simulink model "Pacemaker"  (R2020a)
settings: Solver=FixedStepAuto  StartTime=0.0  StopTime=10.0  FixedStep=1e-3  RelTol=1e-3  EnableMultiTasking=on
undefined symbols (not defined in the file or in its folder): A0, A1, D0, D1, D10, D11, D12, D13, D2, D3, D4, D5, D6, D7, D8, D9, PTA0, PTA1, PTA2, PTB2, PTB23, PTB3, PTB9, PTC16, PTC17, PTC2, PTC3, PTC4, PTD0, PTD1, PTD2, PTD3
libraries: frdmk64flib x21, etargetslib x12, simulink x2
settings Model: ExtModeTrigDuration=5  Creator=Udeep  LastModifiedBy=Udeep
settings OptimizationCC: EnhancedBackFolding=on  PassReuseOutputArgsAs=Individual arguments  ZeroExternalMemoryAtStartup=off  ZeroInternalMemoryAtStartup=off  MaxStackSize=64  OptimizeBlockOrder=speed  DifferentSizesBufferReuse=on  OptimizationCustomize=off  EfficientTunableParamExpr=on
settings DebuggingCC: ParameterTunabilityLossMsg=error
settings HardwareCC: ProdBitPerPointer=32  ProdBitPerSizeT=32  ProdBitPerPtrDiffT=32  ProdLargestAtomicInteger=Long  ProdLargestAtomicFloat=Double  ProdWordSize=32  ProdHWDeviceType=ARM Compatible->ARM Cortex
settings SFSimCC: MATLABDynamicMemAlloc=off
settings RTWCC: SystemTargetFile=ert.tlc  HardwareBoard=NXP FRDM-K64F  TemplateMakefile=ert_default_tmf  Toolchain=GNU Tools for ARM Embedded Processors
settings CodeAppCC: ForceParamTrailComments=on  IgnoreCustomStorageClasses=off  OperatorAnnotations=on  SimulinkDataObjDesc=on  SFDataObjDesc=on  InsertBlockDesc=on
settings ERTTargetCC: TargetLangStandard=C99 (ISO)

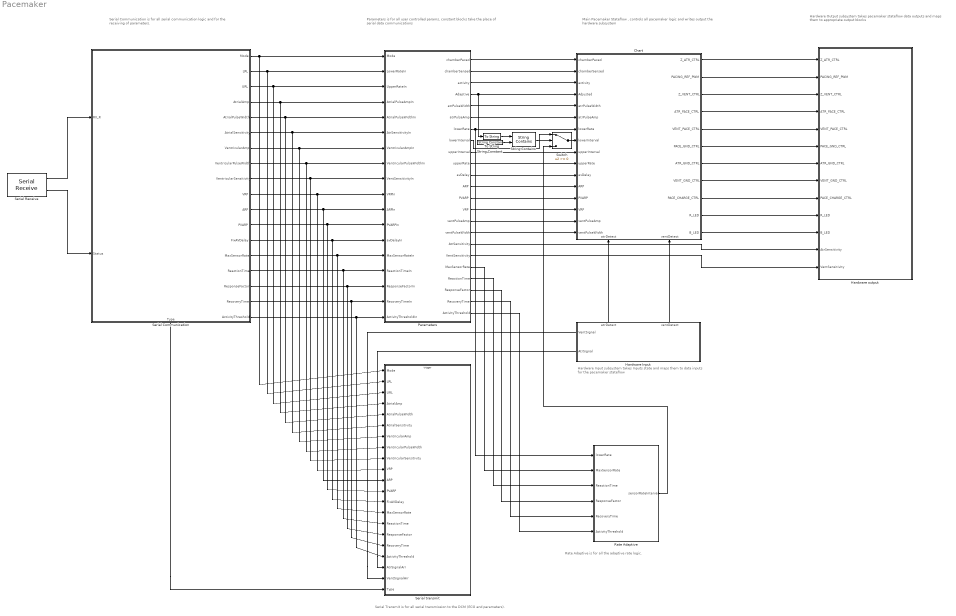
== system Pacemaker ==
  note: Hardware Input subsystem takes Inputs state and maps them to data inputs for the pacemaker stateflow
  note: Hardware Output subsystem takes pacemaker stateflow data outputs and maps them to appropriate output blocks
  note: Main Pacemaker Stateflow , controls all pacemaker logic and writes output the hardware subsystem
  note: Parameters is for all user controlled params, constant blocks take the place of serial data communications
  note: Serial Communication is for all serial communication logic and for the receiving of parameters.
  note: Serial Transmit is for all serial transmission to the DCM (ECG and parameters).
  note: Rate Adaptive is for all the adaptive rate logic.
  Chart : Stateflow chart  TreatAsAtomicUnit=on
      settings: PortSchema="{\"entries\":[{\"content\":{\"sides\":[{\"content\":{\"connectorIds\":[\"In4\",\"In6\",\"In7\",\"In5\",\"In8\",\"In9\",\"In17\",\"In10\",\"In11\",\"In18\",\"In12\",\"In13\",\"In16\",\"In1\",\"In14\",\"In15\"]},\"type\":\"ConnectorPlacement.EquallySpacedRectSide\",\"uuid\":\"0f4bb13e-4f4f-48e2-b63c-32132ec29449\"},{\"content\":{\"connectorIds\":[\"Out1\",\"Out2\",\"Out3\",\"Out4\",\"Out5\",\"Out6\",\"Out7\",\"Out8\",\"Out9\",\"Out10\",\"Out11\"],\"side\":\"RIGHT\"},\"type\":\"ConnectorPlacement.EquallySpacedRectSide\",\"uuid\":\"66676ed7-b2a9-4718-87b6-7ef1563d11ef\"},{\"content\":{\"connectorIds\":[],\"side\":\"TOP\"},\"type\":\"ConnectorPlacement.EquallySpacedRectSide\",\"uuid\":\"f8ed3d2c-017d-4860-9941-e982831d4406\"},{\"content\":{\"connectorIds\":[\"In2\",\"In3\"],\"side\":\"BOTTOM\"},\"type\":\"ConnectorPlacement.EquallySpacedRectSide\",\"uuid\":\"e6b63469-3180-4838-a33b-c03ead75d417\"}]},\"type\":\"ConnectorPlacement.EquallySpacedConnector\",\"uuid\":\"d1db759d-e7ed-4d4b-bc59-5cab093840d4\"}],\"packageUris\":[\"http://schema.mathworks.com/mf0/Connector/19700101\"],\"version\":\"1.0\"}"
  "Hardware Input " : Subsystem
      settings: PortSchema="{\"entries\":[{\"content\":{\"sides\":[{\"content\":{\"connectorIds\":[\"Out3\",\"Out4\"]},\"type\":\"ConnectorPlacement.EquallySpacedRectSide\",\"uuid\":\"9a02dc5a-1337-49ab-8682-c00d401b1034\"},{\"content\":{\"connectorIds\":[],\"side\":\"RIGHT\"},\"type\":\"ConnectorPlacement.EquallySpacedRectSide\",\"uuid\":\"4abd6ab8-13f7-4ac3-81e8-def358981a0b\"},{\"content\":{\"connectorIds\":[\"Out1\",\"Out2\"],\"side\":\"TOP\"},\"type\":\"ConnectorPlacement.EquallySpacedRectSide\",\"uuid\":\"0229585c-8215-4d3e-817f-7000ac7de4ec\"}]},\"type\":\"ConnectorPlacement.EquallySpacedConnector\",\"uuid\":\"98513f05-3720-42c8-8b88-fad36926c18f\"}],\"packageUris\":[\"http://schema.mathworks.com/mf0/Connector/19700101\"],\"version\":\"1.0\"}"
  Hardware output : Subsystem
  Parameters : Subsystem
  Rate Adaptive : Subsystem
  Serial Communication : Stateflow chart  TreatAsAtomicUnit=on
      settings: PortSchema="{\"entries\":[{\"content\":{\"sides\":[{\"content\":{\"connectorIds\":[\"In1\",\"In2\"]},\"type\":\"ConnectorPlacement.EquallySpacedRectSide\",\"uuid\":\"7ad26d3d-dec4-4b7e-9b47-df96273e8372\"},{\"content\":{\"connectorIds\":[\"Out1\",\"Out2\",\"Out3\",\"Out4\",\"Out5\",\"Out16\",\"Out6\",\"Out7\",\"Out17\",\"Out8\",\"Out9\",\"Out10\",\"Out11\",\"Out12\",\"Out13\",\"Out14\",\"Out15\",\"Out18\"],\"side\":\"RIGHT\"},\"type\":\"ConnectorPlacement.EquallySpacedRectSide\",\"uuid\":\"060c4251-7212-4852-acf6-51069082a06b\"},{\"content\":{\"connectorIds\":[],\"side\":\"TOP\"},\"type\":\"ConnectorPlacement.EquallySpacedRectSide\",\"uuid\":\"9bae47f3-580f-4c80-bec3-0b8a7fceacba\"},{\"content\":{\"connectorIds\":[\"Out19\"],\"side\":\"BOTTOM\"},\"type\":\"ConnectorPlacement.EquallySpacedRectSide\",\"uuid\":\"352e057e-9019-4fac-a7bc-ae2107946f91\"}]},\"type\":\"ConnectorPlacement.EquallySpacedConnector\",\"uuid\":\"382a999c-5d0d-4575-8b80-e7cf9b801138\"}],\"packageUris\":[\"http://schema.mathworks.com/mf0/Connector/19700101\"],\"version\":\"1.0\"}"
  Serial Receive : frdmk64flib/Serial Receive  SCIModule=0  Baudrate=uint32(9600)  Parity=None  StopBits=1  HardwareFlowControl=None  ByteOrder=LittleEndian  DataType=uint8  DataLength=40  BlockingMode=off  OutputStatus=on  SampleTime=-1
  Serial transmit : Subsystem  TreatAsAtomicUnit=on
  String Constant : StringConstant  String="\"NONE_AD\""
  String Contains : StringContains
  Switch : Switch
  To String : ToString
  wires:
  Serial Communication/8(VRP) -> Parameters/10(VRPIn), Serial transmit/10(VRP)
  Serial Communication/3(URL) -> Parameters/3(UpperRateIn), Serial transmit/3(URL)
  Parameters/18(VentSensitivity) -> Hardware output/13(VentSensitivity)
  Serial Communication/10(PVARP) -> Parameters/12(PVARPIn), Serial transmit/12(PVARP)
  Serial Communication/11(FixAVDelay) -> Parameters/13(avDelayIn), Serial transmit/13(FixAVDelay)
  Chart/6(PACE_GND_CTRL) -> Hardware output/6(PACE_GND_CTRL)
  Serial Communication/16(AtrialSensitivity) -> Parameters/6(AtrSensitivityIn), Serial transmit/6(AtrialSensitivity)
  Serial Communication/2(LRL) -> Parameters/2(LowerRateIn), Serial transmit/2(LRL)
  Serial Receive/1 -> Serial Communication/1(RX_R)
  Serial Communication/4(AtrialAmp) -> Parameters/4(AtrialPulseAmpIn), Serial transmit/4(AtrialAmp)
  Serial Receive/2 -> Serial Communication/2(Status)
  Serial Communication/1(Mode) -> Parameters/1(Mode), Serial transmit/1(Mode)
  Chart/5(VENT_PACE_CTRL) -> Hardware output/5(VENT_PACE_CTRL)
  Serial Communication/7(VentricularPulseWidth) -> Parameters/8(VentricularPulseWidthIn), Serial transmit/8(VentricularPulseWidth)
  Chart/9(PACE_CHARGE_CTRL) -> Hardware output/9(PACE_CHARGE_CTRL)
  Parameters/12(ARP) -> Chart/13(ARP)
  Parameters/4(Adaptive) -> To String/1, Chart/5(Adjusted)
  Parameters/17(AtrSensitivity) -> Hardware output/12(AtrSensitivity)
  Serial Communication/5(AtrialPulseWidth) -> Parameters/5(AtrialPulseWidthIn), Serial transmit/5(AtrialPulseWidth)
  Serial Communication/9(ARP) -> Parameters/11(ARPIn), Serial transmit/11(ARP)
  Chart/2(PACING_REF_PWM) -> Hardware output/2(PACING_REF_PWM)
  Parameters/6(atrPulseAmp) -> Chart/9(atrPulseAmp)
  Parameters/5(atrPulseWidth) -> Chart/8(atrPulseWidth)
  "Hardware Input "/2(ventDetect) -> Chart/3(ventDetect)
  Parameters/10(upperRate) -> Chart/18(upperRate)
  Parameters/7(lowerRate) -> Rate Adaptive/1(lowerRate), Chart/17(lowerRate)
  Chart/1(Z_ATR_CTRL) -> Hardware output/1(Z_ATR_CTRL)
  "Hardware Input "/1(atrDetect) -> Chart/2(atrDetect)
  Parameters/13(PVARP) -> Chart/16(PVARP)
  Chart/4(ATR_PACE_CTRL) -> Hardware output/4(ATR_PACE_CTRL)
  Chart/3(Z_VENT_CTRL) -> Hardware output/3(Z_VENT_CTRL)
  Parameters/1(chamberPaced) -> Chart/4(chamberPaced)
  Chart/7(ATR_GND_CTRL) -> Hardware output/7(ATR_GND_CTRL)
  Parameters/11(avDelay) -> Chart/12(avDelay)
  Parameters/3(activity) -> Chart/7(activity)
  Parameters/2(chamberSensed) -> Chart/6(chamberSensed)
  Chart/8(VENT_GND_CTRL) -> Hardware output/8(VENT_GND_CTRL)
  Parameters/9(upperInterval) -> Chart/11(upperInterval)
  Parameters/14(VRP) -> Chart/1(VRP)
  Serial Communication/6(VentricularAmp) -> Parameters/7(VentricularAmpIn), Serial transmit/7(VentricularAmp)
  Serial Communication/17(VentricularSensitivity) -> Parameters/9(VentSensitivityIn), Serial transmit/9(VentricularSensitivity)
  Serial Communication/12(MaxSensorRate) -> Parameters/14(MaxSensorRateIn), Serial transmit/14(MaxSensorRate)
  Serial Communication/14(ResponseFactor) -> Parameters/16(ResponseFactorIn), Serial transmit/16(ResponseFactor)
  Serial Communication/15(RecoveryTime) -> Parameters/17(RecoveryTimeIn), Serial transmit/17(RecoveryTime)
  Serial Communication/18(ActivityThreshold) -> Parameters/18(ActivityThresholdIn), Serial transmit/18(ActivityThreshold)
  Parameters/15(ventPulseAmp) -> Chart/14(ventPulseAmp)
  Parameters/16(ventPulseWidth) -> Chart/15(ventPulseWidth)
  "Hardware Input "/4(AtrSignal) -> Serial transmit/19(AtrSignalArr)
  "Hardware Input "/3(VentSignal) -> Serial transmit/20(VentSignalArr)
  Serial Communication/13(ReactionTime) -> Parameters/15(ReactionTimeIn), Serial transmit/15(ReactionTime)
  Serial Communication/19(Type) -> Serial transmit/21(Type)
  Rate Adaptive/1(sensorRateInterval) -> Switch/3
  Parameters/8(lowerInterval) -> Switch/1
  String Constant/1 -> String Contains/2
  String Contains/1 -> Switch/2
  Switch/1 -> Chart/10(lowerInterval)
  Chart/10(R_LED) -> Hardware output/10(R_LED)
  Chart/11(B_LED) -> Hardware output/11(B_LED)
  Parameters/19(MaxSensorRate) -> Rate Adaptive/2(MaxSensorRate)
  Parameters/20(ReactionTime) -> Rate Adaptive/3(ReactionTime)
  Parameters/21(ResponseFactor) -> Rate Adaptive/4(ResponseFactor)
  Parameters/22(RecoveryTime) -> Rate Adaptive/5(RecoveryTime)
  Parameters/23(ActivityThreshold) -> Rate Adaptive/6(ActivityThreshold)
  To String/1 -> String Contains/1

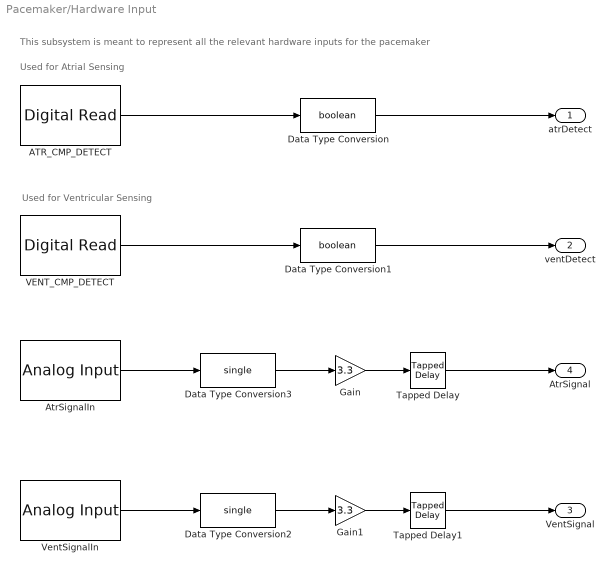
== system Pacemaker/Hardware Input  ==
  note: This subsystem is meant to represent all the relevant hardware inputs for the pacemaker
  note: Used for Atrial Sensing
  note: Used for Ventricular Sensing
  ATR_CMP_DETECT : frdmk64flib/Digital Read  Whichpin=PTC16 (D0)  SampleTime=-1
  AtrSignalIn : frdmk64flib/Analog Input  Whichpin=PTB2 (A0)  SampleTime=-1
  Data Type Conversion : DataTypeConversion  OutDataTypeStr=boolean  RndMeth=Round
  Data Type Conversion1 : DataTypeConversion  OutDataTypeStr=boolean  RndMeth=Round
  Data Type Conversion2 : DataTypeConversion  OutDataTypeStr=single  RndMeth=Nearest
  Data Type Conversion3 : DataTypeConversion  OutDataTypeStr=single  RndMeth=Nearest
  Gain : Gain  Gain=3.3
  Gain1 : Gain  Gain=3.3
  Tapped Delay : simulink/Discrete/Tapped Delay  vinit=0.0  samptime=0.002  NumDelays=9  DelayOrder=Oldest  includeCurrent=on
  Tapped Delay1 : simulink/Discrete/Tapped Delay  vinit=0.0  samptime=0.002  NumDelays=9  DelayOrder=Oldest  includeCurrent=on
  VENT_CMP_DETECT : frdmk64flib/Digital Read  Whichpin=PTC17 (D1)  SampleTime=-1
  VentSignalIn : frdmk64flib/Analog Input  Whichpin=PTB3 (A1)  SampleTime=-1
  atrDetect : Outport  OutDataTypeStr=boolean
  ventDetect : Outport  Port=2  OutDataTypeStr=boolean
  VentSignal : Outport  Port=3
  AtrSignal : Outport  Port=4
  wires:
  Data Type Conversion/1 -> atrDetect/1
  VENT_CMP_DETECT/1 -> Data Type Conversion1/1
  Data Type Conversion1/1 -> ventDetect/1
  ATR_CMP_DETECT/1 -> Data Type Conversion/1
  Data Type Conversion3/1 -> Gain/1
  VentSignalIn/1 -> Data Type Conversion2/1
  AtrSignalIn/1 -> Data Type Conversion3/1
  Data Type Conversion2/1 -> Gain1/1
  Gain/1 -> Tapped Delay/1
  Tapped Delay/1 -> AtrSignal/1
  Gain1/1 -> Tapped Delay1/1
  Tapped Delay1/1 -> VentSignal/1

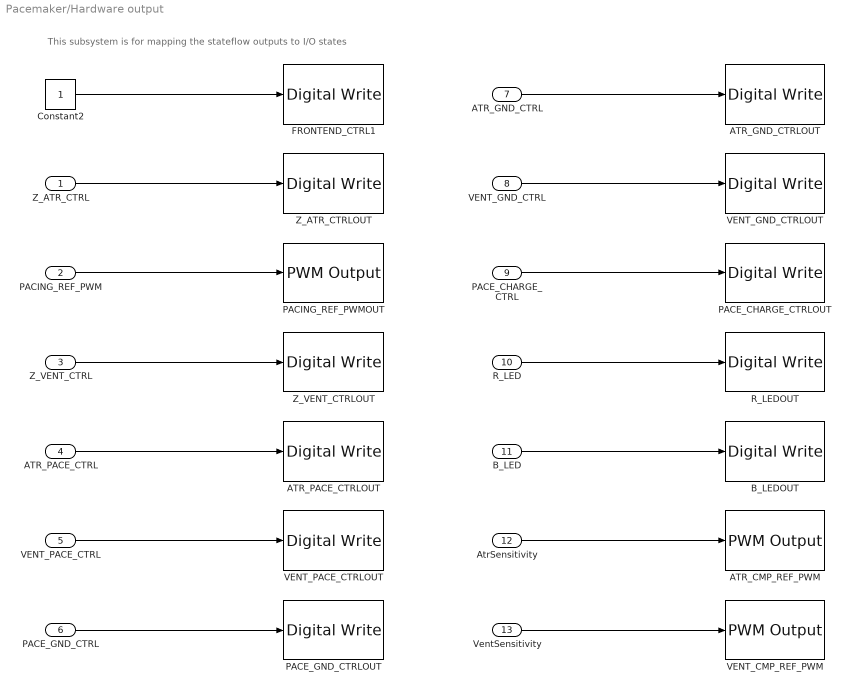
== system Pacemaker/Hardware output ==
  note: This subsystem is for mapping the stateflow outputs to I/O states
  Z_ATR_CTRL : Inport
  PACING_REF_PWM : Inport  Port=2
  Z_VENT_CTRL : Inport  Port=3
  ATR_PACE_CTRL : Inport  Port=4
  VENT_PACE_CTRL : Inport  Port=5
  PACE_GND_CTRL : Inport  Port=6
  ATR_GND_CTRL : Inport  Port=7
  VENT_GND_CTRL : Inport  Port=8
  PACE_CHARGE_CTRL : Inport  Port=9
  R_LED : Inport  Port=10
  B_LED : Inport  Port=11
  AtrSensitivity : Inport  Port=12
  VentSensitivity : Inport  Port=13
  ATR_CMP_REF_PWM : frdmk64flib/PWM Output  Whichpin=PTC2 (D6)  InitialFrequency=2000  InitialDutyCycle=0
  ATR_GND_CTRLOUT : frdmk64flib/Digital Write  Whichpin=PTD2 (D11)
  ATR_PACE_CTRLOUT : frdmk64flib/Digital Write  Whichpin=PTA0 (D8)
  B_LEDOUT : frdmk64flib/Digital Write  Whichpin=BLUE_LED
  Constant2 : Constant
  FRONTEND_CTRL1 : frdmk64flib/Digital Write  Whichpin=PTD1 (D13)
  PACE_CHARGE_CTRLOUT : frdmk64flib/Digital Write  Whichpin=PTB9 (D2)
  PACE_GND_CTRLOUT : frdmk64flib/Digital Write  Whichpin=PTD0 (D10)
  PACING_REF_PWMOUT : frdmk64flib/PWM Output  Whichpin=PTA2 (D5)  InitialFrequency=2000  InitialDutyCycle=0
  R_LEDOUT : frdmk64flib/Digital Write  Whichpin=RED_LED
  VENT_CMP_REF_PWM : frdmk64flib/PWM Output  Whichpin=PTA1 (D3)  InitialFrequency=2000  InitialDutyCycle=0
  VENT_GND_CTRLOUT : frdmk64flib/Digital Write  Whichpin=PTD3 (D12)
  VENT_PACE_CTRLOUT : frdmk64flib/Digital Write  Whichpin=PTC4 (D9)
  Z_ATR_CTRLOUT : frdmk64flib/Digital Write  Whichpin=PTB23 (D4)
  Z_VENT_CTRLOUT : frdmk64flib/Digital Write  Whichpin=PTC3 (D7)
  wires:
  Constant2/1 -> FRONTEND_CTRL1/1
  Z_ATR_CTRL/1 -> Z_ATR_CTRLOUT/1
  PACING_REF_PWM/1 -> PACING_REF_PWMOUT/1
  Z_VENT_CTRL/1 -> Z_VENT_CTRLOUT/1
  ATR_PACE_CTRL/1 -> ATR_PACE_CTRLOUT/1
  VENT_PACE_CTRL/1 -> VENT_PACE_CTRLOUT/1
  PACE_GND_CTRL/1 -> PACE_GND_CTRLOUT/1
  ATR_GND_CTRL/1 -> ATR_GND_CTRLOUT/1
  VENT_GND_CTRL/1 -> VENT_GND_CTRLOUT/1
  PACE_CHARGE_CTRL/1 -> PACE_CHARGE_CTRLOUT/1
  R_LED/1 -> R_LEDOUT/1
  B_LED/1 -> B_LEDOUT/1
  AtrSensitivity/1 -> ATR_CMP_REF_PWM/1
  VentSensitivity/1 -> VENT_CMP_REF_PWM/1

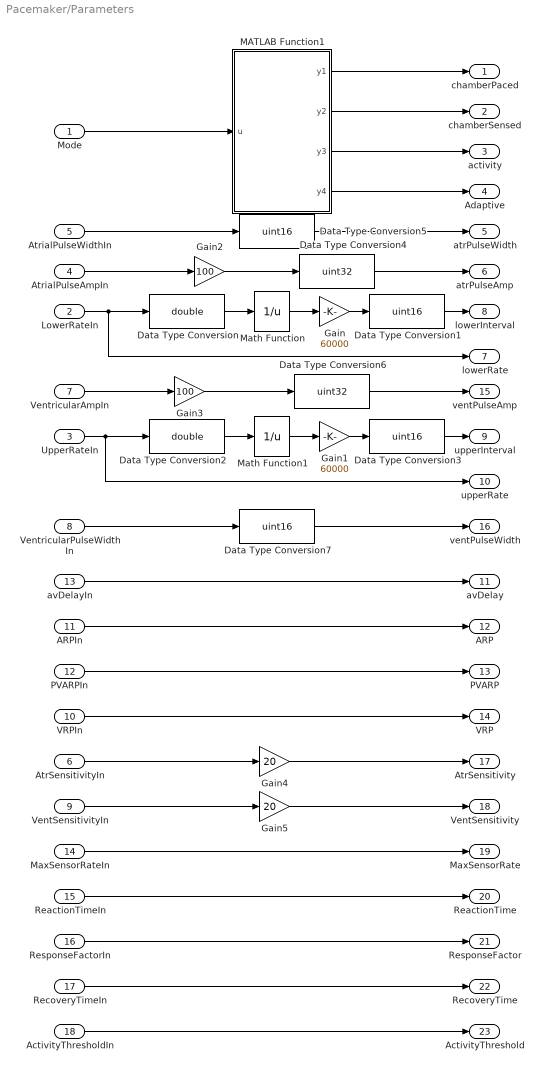
== system Pacemaker/Parameters ==
  Mode : Inport
  LowerRateIn : Inport  Port=2  Unit=ppm
  UpperRateIn : Inport  Port=3  Unit=ppm
  AtrialPulseAmpIn : Inport  Port=4
  AtrialPulseWidthIn : Inport  Port=5
  AtrSensitivityIn : Inport  Port=6
  VentricularAmpIn : Inport  Port=7
  VentricularPulseWidthIn : Inport  Port=8
  VentSensitivityIn : Inport  Port=9
  VRPIn : Inport  Port=10
  ARPIn : Inport  Port=11
  PVARPIn : Inport  Port=12
  avDelayIn : Inport  Port=13  Unit=ms
  MaxSensorRateIn : Inport  Port=14
  ReactionTimeIn : Inport  Port=15
  ResponseFactorIn : Inport  Port=16
  RecoveryTimeIn : Inport  Port=17
  ActivityThresholdIn : Inport  Port=18
  Data Type Conversion : DataTypeConversion  OutDataTypeStr=double
  Data Type Conversion1 : DataTypeConversion  OutDataTypeStr=uint16
  Data Type Conversion2 : DataTypeConversion  OutDataTypeStr=double
  Data Type Conversion3 : DataTypeConversion  OutDataTypeStr=uint16
  Data Type Conversion4 : DataTypeConversion  OutDataTypeStr=uint32  RndMeth=Round
  Data Type Conversion5 : DataTypeConversion  OutDataTypeStr=uint16  RndMeth=Nearest
  Data Type Conversion6 : DataTypeConversion  OutDataTypeStr=uint32  RndMeth=Round
  Data Type Conversion7 : DataTypeConversion  OutDataTypeStr=uint16  RndMeth=Nearest
  Gain : Gain  Gain=60000  OutDataTypeStr=double
  Gain1 : Gain  Gain=60000  OutDataTypeStr=double
  Gain2 : Gain  Gain=100
  Gain3 : Gain  Gain=100
  Gain4 : Gain  Gain=20
  Gain5 : Gain  Gain=20
  MATLAB Function1 : MATLAB Function  TreatAsAtomicUnit=on
  Math Function : Math  Operator=reciprocal  SaturateOnIntegerOverflow=on
  Math Function1 : Math  Operator=reciprocal  SaturateOnIntegerOverflow=on
  chamberPaced : Outport  OutDataTypeStr=Enum: ChamberPaced
  chamberSensed : Outport  Port=2  OutDataTypeStr=Enum: ChamberSensed
  activity : Outport  Port=3  OutDataTypeStr=Enum: Activity
  Adaptive : Outport  Port=4  OutDataTypeStr=Enum: Adaptive
  atrPulseWidth : Outport  Port=5  Unit=ms
  atrPulseAmp : Outport  Port=6  Unit=mV
  lowerRate : Outport  Port=7  Unit=ppm
  lowerInterval : Outport  Port=8  Unit=ms
  upperInterval : Outport  Port=9  Unit=ms
  upperRate : Outport  Port=10  Unit=ppm
  avDelay : Outport  Port=11
  ARP : Outport  Port=12
  PVARP : Outport  Port=13
  VRP : Outport  Port=14
  ventPulseAmp : Outport  Port=15
  ventPulseWidth : Outport  Port=16
  AtrSensitivity : Outport  Port=17
  VentSensitivity : Outport  Port=18
  MaxSensorRate : Outport  Port=19
  ReactionTime : Outport  Port=20
  ResponseFactor : Outport  Port=21
  RecoveryTime : Outport  Port=22
  ActivityThreshold : Outport  Port=23
  wires:
  AtrialPulseAmpIn/1 -> Gain2/1
  avDelayIn/1 -> avDelay/1
  Math Function/1 -> Gain/1
  Gain/1 -> Data Type Conversion1/1
  LowerRateIn/1 -> lowerRate/1, Data Type Conversion/1
  Math Function1/1 -> Gain1/1
  UpperRateIn/1 -> upperRate/1, Data Type Conversion2/1
  Gain1/1 -> Data Type Conversion3/1
  AtrSensitivityIn/1 -> Gain4/1
  VentSensitivityIn/1 -> Gain5/1
  VRPIn/1 -> VRP/1
  PVARPIn/1 -> PVARP/1
  ARPIn/1 -> ARP/1
  Data Type Conversion/1 -> Math Function/1
  Data Type Conversion1/1 -> lowerInterval/1
  Data Type Conversion2/1 -> Math Function1/1
  Data Type Conversion3/1 -> upperInterval/1
  Gain2/1 -> Data Type Conversion4/1
  Data Type Conversion4/1 -> atrPulseAmp/1
  MATLAB Function1/1(y1) -> chamberPaced/1
  MATLAB Function1/2(y2) -> chamberSensed/1
  MATLAB Function1/3(y3) -> activity/1
  MATLAB Function1/4(y4) -> Adaptive/1
  Mode/1 -> MATLAB Function1/1(u)
  AtrialPulseWidthIn/1 -> Data Type Conversion5/1
  Data Type Conversion5/1 -> atrPulseWidth/1
  Data Type Conversion6/1 -> ventPulseAmp/1
  Gain3/1 -> Data Type Conversion6/1
  VentricularAmpIn/1 -> Gain3/1
  VentricularPulseWidthIn/1 -> Data Type Conversion7/1
  Data Type Conversion7/1 -> ventPulseWidth/1
  Gain4/1 -> AtrSensitivity/1
  Gain5/1 -> VentSensitivity/1
  MaxSensorRateIn/1 -> MaxSensorRate/1
  ReactionTimeIn/1 -> ReactionTime/1
  ResponseFactorIn/1 -> ResponseFactor/1
  RecoveryTimeIn/1 -> RecoveryTime/1
  ActivityThresholdIn/1 -> ActivityThreshold/1

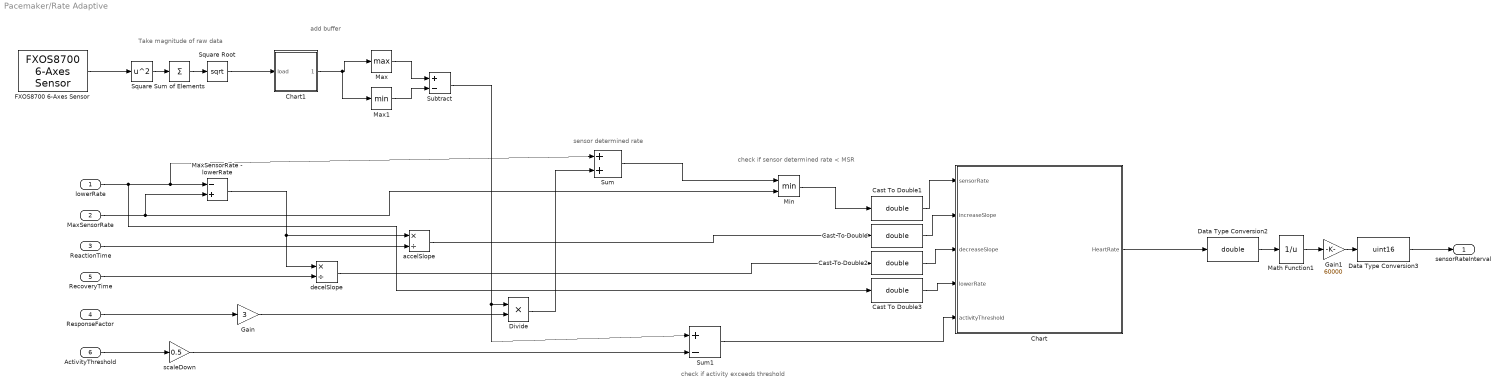
== system Pacemaker/Rate Adaptive ==
  note: check if activity exceeds threshold
  note: Take magnitude of raw data
  note: add buffer
  note: check if sensor determined rate < MSR
  note: sensor determined rate
  lowerRate : Inport
  MaxSensorRate : Inport  Port=2
  ReactionTime : Inport  Port=3
  ResponseFactor : Inport  Port=4
  RecoveryTime : Inport  Port=5
  ActivityThreshold : Inport  Port=6
  Cast To Double{,1..3} (4 alike) : DataTypeConversion  OutDataTypeStr=double
  Chart : Stateflow chart  TreatAsAtomicUnit=on
      settings: PortSchema="{\"entries\":[{\"content\":{\"sides\":[{\"content\":{\"connectorIds\":[\"In1\",\"In2\",\"In3\",\"In5\",\"In4\"]},\"type\":\"ConnectorPlacement.EquallySpacedRectSide\",\"uuid\":\"280d3624-73d1-46b8-bef9-6b152ff520d0\"},{\"content\":{\"connectorIds\":[\"Out1\"],\"side\":\"RIGHT\"},\"type\":\"ConnectorPlacement.EquallySpacedRectSide\",\"uuid\":\"ca231bc9-092d-4f04-92da-0e5e1126d83a\"},{\"content\":{\"connectorIds\":[],\"side\":\"TOP\"},\"type\":\"ConnectorPlacement.EquallySpacedRectSide\",\"uuid\":\"4925a7c4-ebdf-49b7-bb10-6299dcbd8d2b\"}]},\"type\":\"ConnectorPlacement.EquallySpacedConnector\",\"uuid\":\"ff1ab066-13d6-46ea-96f3-1f62e14f4410\"}],\"packageUris\":[\"http://schema.mathworks.com/mf0/Connector/19700101\"],\"version\":\"1.0\"}"
  Chart1 : Stateflow chart  TreatAsAtomicUnit=on
  Data Type Conversion2 : DataTypeConversion  OutDataTypeStr=double
  Data Type Conversion3 : DataTypeConversion  OutDataTypeStr=uint16
  Divide : Product  Inputs=**
  FXOS8700 6-Axes Sensor : frdmk64flib/FXOS8700 6-Axes Sensor  Activesensor=Accelerometer only  ODR=800Hz  HybridODR=400Hz  Accelfullrange=-4g to +4g  SampleTime=-1
  Gain : Gain  Gain=3
  Gain1 : Gain  Gain=60000  OutDataTypeStr=double
  Math Function1 : Math  Operator=reciprocal  SaturateOnIntegerOverflow=on
  Max : MinMax  Function=max
  Max1 : MinMax
  MaxSensorRate - lowerRate : Sum  Inputs=-+
  Min : MinMax  Inputs=2
  Square : Math  Operator=square  SaturateOnIntegerOverflow=on
  Square Root : Sqrt  SaturateOnIntegerOverflow=on
  Subtract : Sum  Inputs=+-
  Sum : Sum  Inputs=|++
  Sum of Elements : Sum  Inputs=+
  Sum1 : Sum  Inputs=|+-
  accelSlope : Product  Inputs=*/
  decelSlope : Product  Inputs=*/
  scaleDown : Gain  Gain=0.5
  sensorRateInterval : Outport
  wires:
  FXOS8700 6-Axes Sensor/1 -> Square/1
  Square/1 -> Sum of Elements/1
  Sum of Elements/1 -> Square Root/1
  ActivityThreshold/1 -> scaleDown/1
  MaxSensorRate/1 -> Min/2, MaxSensorRate - lowerRate/2
  scaleDown/1 -> Sum1/2
  ResponseFactor/1 -> Gain/1
  Divide/1 -> Sum/2
  MaxSensorRate - lowerRate/1 -> decelSlope/1, accelSlope/1
  ReactionTime/1 -> accelSlope/2
  Sum/1 -> Min/1
  Data Type Conversion2/1 -> Math Function1/1
  Math Function1/1 -> Gain1/1
  Chart/1(HeartRate) -> Data Type Conversion2/1
  Gain1/1 -> Data Type Conversion3/1
  Data Type Conversion3/1 -> sensorRateInterval/1
  Min/1 -> Cast To Double1/1
  accelSlope/1 -> Cast To Double/1
  lowerRate/1 -> Cast To Double3/1, Sum/1, MaxSensorRate - lowerRate/1
  Square Root/1 -> Chart1/1(load)
  Subtract/1 -> Sum1/1, Divide/1
  Sum1/1 -> Chart/4(activityThreshold)
  Cast To Double/1 -> Chart/2(increaseSlope)
  Cast To Double1/1 -> Chart/1(sensorRate)
  Cast To Double3/1 -> Chart/5(lowerRate)
  Cast To Double2/1 -> Chart/3(decreaseSlope)
  decelSlope/1 -> Cast To Double2/1
  RecoveryTime/1 -> decelSlope/2
  Gain/1 -> Divide/2
  Chart1/1(Activity) -> Max1/1, Max/1
  Max/1 -> Subtract/1
  Max1/1 -> Subtract/2

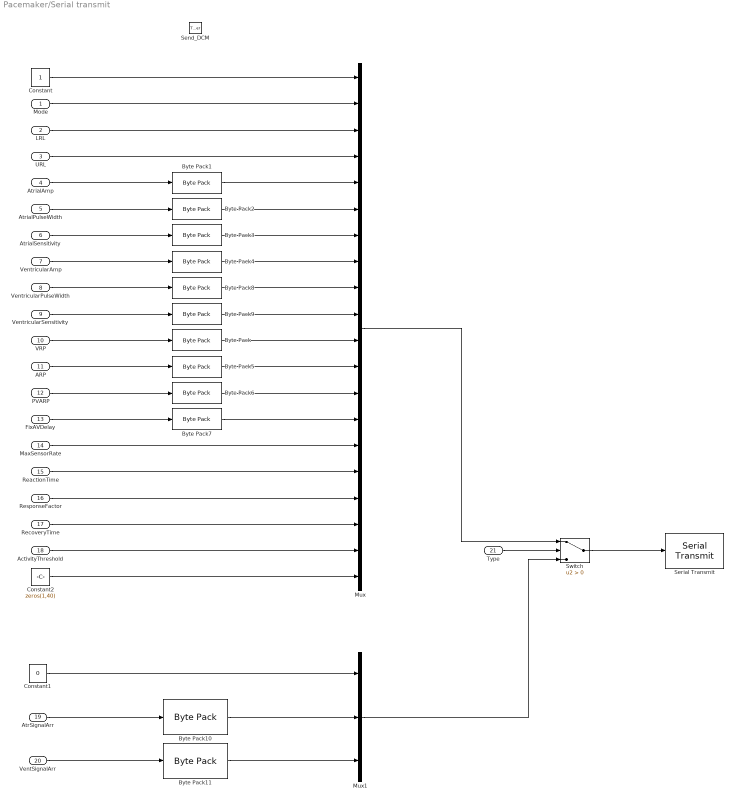
== system Pacemaker/Serial transmit ==
  Mode : Inport  OutDataTypeStr=uint8
  LRL : Inport  Port=2  OutDataTypeStr=uint8
  URL : Inport  Port=3  OutDataTypeStr=uint8
  AtrialAmp : Inport  Port=4  OutDataTypeStr=single
  AtrialPulseWidth : Inport  Port=5  OutDataTypeStr=single
  AtrialSensitivity : Inport  Port=6  OutDataTypeStr=single
  VentricularAmp : Inport  Port=7  OutDataTypeStr=single
  VentricularPulseWidth : Inport  Port=8  OutDataTypeStr=single
  VentricularSensitivity : Inport  Port=9  OutDataTypeStr=single
  VRP : Inport  Port=10  OutDataTypeStr=uint16
  ARP : Inport  Port=11  OutDataTypeStr=uint16
  PVARP : Inport  Port=12  OutDataTypeStr=uint16
  FixAVDelay : Inport  Port=13  OutDataTypeStr=uint16
  MaxSensorRate : Inport  Port=14  OutDataTypeStr=uint8
  ReactionTime : Inport  Port=15  OutDataTypeStr=uint8
  ResponseFactor : Inport  Port=16  OutDataTypeStr=uint8
  RecoveryTime : Inport  Port=17  OutDataTypeStr=uint8
  ActivityThreshold : Inport  Port=18  OutDataTypeStr=uint8
  AtrSignalArr : Inport  Port=19  OutDataTypeStr=single
  VentSignalArr : Inport  Port=20  OutDataTypeStr=single
  Type : Inport  Port=21  OutDataTypeStr=uint8
  Send_DCM : TriggerPort  TriggerType=function-call  IsSimulinkFunction=on  FunctionName=Send_DCM  VariantControl=Variant
  Byte Pack{,5..7} (4 alike) : etargetslib/Byte Pack  datatypes={'uint16'}  byteAlign=1
  Byte Pack{1..4,8..11} (8 alike) : etargetslib/Byte Pack  datatypes={'single'}  byteAlign=1
  Constant : Constant  OutDataTypeStr=uint8
  Constant1 : Constant  Value=0  OutDataTypeStr=uint8
  Constant2 : Constant  Value=zeros(1,40)  OutDataTypeStr=uint8
  Mux : Mux  Inputs=20
  Mux1 : Mux  Inputs=3
  Serial Transmit : frdmk64flib/Serial Transmit  SCIModule=0  Baudrate=uint32(9600)  Parity=None  StopBits=1  HardwareFlowControl=None  ByteOrder=LittleEndian  BlockingMode=on  OutputStatus=off
  Switch : Switch  Criteria=u2 > Threshold
  wires:
  Constant/1 -> Mux/1
  Mode/1 -> Mux/2
  LRL/1 -> Mux/3
  URL/1 -> Mux/4
  AtrialAmp/1 -> Byte Pack1/1
  Byte Pack1/1 -> Mux/5
  AtrialPulseWidth/1 -> Byte Pack2/1
  AtrialSensitivity/1 -> Byte Pack3/1
  VentricularAmp/1 -> Byte Pack4/1
  VentricularPulseWidth/1 -> Byte Pack8/1
  VentricularSensitivity/1 -> Byte Pack9/1
  VRP/1 -> Byte Pack/1
  ARP/1 -> Byte Pack5/1
  PVARP/1 -> Byte Pack6/1
  FixAVDelay/1 -> Byte Pack7/1
  Byte Pack2/1 -> Mux/6
  Byte Pack3/1 -> Mux/7
  Byte Pack4/1 -> Mux/8
  Byte Pack8/1 -> Mux/9
  Byte Pack9/1 -> Mux/10
  Byte Pack/1 -> Mux/11
  Byte Pack5/1 -> Mux/12
  Byte Pack6/1 -> Mux/13
  Byte Pack7/1 -> Mux/14
  MaxSensorRate/1 -> Mux/15
  ReactionTime/1 -> Mux/16
  ResponseFactor/1 -> Mux/17
  RecoveryTime/1 -> Mux/18
  ActivityThreshold/1 -> Mux/19
  Byte Pack10/1 -> Mux1/2
  VentSignalArr/1 -> Byte Pack11/1
  Constant1/1 -> Mux1/1
  Byte Pack11/1 -> Mux1/3
  AtrSignalArr/1 -> Byte Pack10/1
  Mux/1 -> Switch/1
  Type/1 -> Switch/2
  Mux1/1 -> Switch/3
  Switch/1 -> Serial Transmit/1
  Constant2/1 -> Mux/20

== matlab function Pacemaker/Parameters/MATLAB Function1 ==
  data: u input; y1 output; y2 output; y3 output; y4 output
function [y1,y2,y3,y4] = fcn(u)
    y1 = ChamberPaced.ATRIUM_P;
    y2 = ChamberSensed.NONE_S;
    y3 = Activity.NONE_A;
    y4 = Adaptive.NONE_AD;
    if(u == 0)
       y1 = ChamberPaced.ATRIUM_P;
       y2 = ChamberSensed.NONE_S;
       y3 = Activity.NONE_A;
       y4 = Adaptive.NONE_AD;
    elseif(u == 1)
       y1 = ChamberPaced.ATRIUM_P;
       y2 = ChamberSensed.ATRIUM_S;
       y3 = Activity.INHIBITED_A;
       y4 = Adaptive.NONE_AD;
    elseif(u == 2)
       y1 = ChamberPaced.ATRIUM_P;
       y2 = ChamberSensed.NONE_S;
       y3 = Activity.NONE_A;
       y4 = Adaptive.RATE_AD;
    elseif(u == 3)
       y1 = ChamberPaced.ATRIUM_P;
       y2 = ChamberSensed.ATRIUM_S;
       y3 = Activity.INHIBITED_A;
       y4 = Adaptive.RATE_AD;
    elseif(u == 4)
       y1 = ChamberPaced.VENTRICLE_P;
       y2 = ChamberSensed.NONE_S;
       y3 = Activity.NONE_A;
       y4 = Adaptive.NONE_AD;
    elseif(u == 5)
       y1 = ChamberPaced.VENTRICLE_P;
       y2 = ChamberSensed.VENTRICLE_S;
       y3 = Activity.INHIBITED_A;
       y4 = Adaptive.NONE_AD;
    elseif(u == 6)
       y1 = ChamberPaced.VENTRICLE_P;
       y2 = ChamberSensed.NONE_S;
       y3 = Activity.NONE_A;
       y4 = Adaptive.RATE_AD;
    elseif(u == 7)
       y1 = ChamberPaced.VENTRICLE_P;
       y2 = ChamberSensed.VENTRICLE_S;
       y3 = Activity.INHIBITED_A;
       y4 = Adaptive.RATE_AD;
    elseif(u == 8)
       y1 = ChamberPaced.DUAL_P;
       y2 = ChamberSensed.NONE_S;
       y3 = Activity.NONE_A;
       y4 = Adaptive.NONE_AD;
    elseif(u == 9)
       y1 = ChamberPaced.DUAL_P;
       y2 = ChamberSensed.NONE_S;
       y3 = Activity.NONE_A;
       y4 = Adaptive.RATE_AD;
    elseif(u == 10)
       y1 = ChamberPaced.DUAL_P;
       y2 = ChamberSensed.DUAL_S;
       y3 = Activity.DUAL_A;
       y4 = Adaptive.RATE_AD;
    end
end

== stateflow chart Pacemaker/Chart ==
  note: Init
      | This state is meant for any boot-up operations that need to occur once before normal operation.Intial pin configurations and the capacitor is pre-charged here.
  state INIT
    Z_ATR_CTRL = false;
    Z_VENT_CTRL = false;
    % selecting correct initial pulse amplitude
    if chamberPaced == ChamberPaced.VENTRICLE_P
    pulseAmp = ventPulseAmp;
    else
    pulseAmp = atrPulseAmp;
    end
    PACING_REF_PWM = (pulseAmp/5);
    ATR_PACE_CTRL = false;
    VENT_PACE_CTRL = false;
    PACE_GND_CTRL = true;
    ATR_GND_CTRL = false;
    VENT_GND_CTRL = false;
    PACE_CHARGE_CTRL = true;
    R_LED = false; %testing pin
    B_LED = false; %testing pin
  state Sense
    note: Loops back for sensed case in inhibited
    state Default
    note: Default exists to constantly check if the mode is the same or is changed.
    note: For DXXX or XDXX or AXXX or XAXX modes
    note: For VXXX or XVXX modes
    note: Loops back for sensed case in inhibited
    state Ventricle
      state Default
        ActiveChamber = 2;
        %Update pace params to chamber
        pulseWidth = ventPulseWidth
        pulseAmp = ventPulseAmp
      note: Sets the active chamber, which directs where to pace
          | 1 = Atrium
          | 2 = Ventrical
      state Inhibited_VRP
        %Waits for VRP before sensing
      state None
        %Wait for a time then pace
      state Inhibited
        %checks if the heart paced
      state PaceSend
        %Sends to Pace
        send(paceStart)
      (default) -> Sense.Ventricle.Default
      Sense.Ventricle.Default -> (junction 147)
      (junction 147) -> Inhibited_VRP [order 1] : [activity == Activity.INHIBITED_A]
      (junction 147) -> Sense.Ventricle.None [order 2] : [activity == Activity.NONE_A]
      Inhibited_VRP -> Inhibited : after(VRP-pulseWidth,msec)
      Sense.Ventricle.None -> Sense.Ventricle.PaceSend [order 1] : [after(avDelay,msec) && dualSense(chamberPaced,chamberSensed)]
      Sense.Ventricle.None -> Sense.Ventricle.PaceSend [order 2] : after(lowerInterval-pulseWidth,msec)
      Inhibited -> Sense.Ventricle.PaceSend [order 1] : after(lowerInterval-VRP+12,msec)
    note: Fired from Pace after a pulse is sent and if ventricular sensing still needs to occur for XDXX and DXXX modes
    state Atrium
      state Default
        ActiveChamber = 1;
        %Update pace params to chamber
        pulseWidth = atrPulseWidth
        pulseAmp = atrPulseAmp
      note: Sets the active chamber, which directs where to pace
          | 1 = Atrium
          | 2 = Ventrical
      note: Junction detects the activity modes
      state Tiggered
        %code for detecting Pwave
        %if found executes
        %send(V_PaceBypass)
        %meant for Dual modes
      state Inhibited_ARP
        %Waits for ARP before sensing
      state None
        %Wait then pace
      state InhibitedSense
        %checks if the heart paced
      state PaceSend
        %sends to pace
        send(paceStart)
      (default) -> Sense.Atrium.Default
      Sense.Atrium.Default -> (junction 135)
      (junction 135) -> Tiggered [order 1] : [activity == Activity.DUAL_A]
      (junction 135) -> Sense.Atrium.None [order 2] : [activity == Activity.NONE_A]
      (junction 135) -> Inhibited_ARP [order 3] : [activity == Activity.INHIBITED_A]
      Inhibited_ARP -> InhibitedSense : after(ARP-pulseWidth,msec)
      Sense.Atrium.None -> Sense.Atrium.PaceSend : after(lowerInterval,msec)
      InhibitedSense -> Sense.Atrium.PaceSend [order 1] : after(lowerInterval-ARP+10,msec)
    note: Senses the Atrium
    note: Senses the Ventricle
    note: Function to validate transistion between Default and Ventricle
    note: Function to validate transistion between Default and Atrium
    InhibitedSense -> Sense.Default [order 2] : [atrDetect == true]/{after(pulseWidth+10,msec)}
    Inhibited -> Sense.Default [order 2] : [ventDetect == true]/{after(pulseWidth+10,msec)}
    (default) -> Sense.Default
    Sense.Default -> Ventricle [order 1] : [ventSense(chamberPaced,chamberSensed)==1]
    Sense.Default -> Atrium [order 2] : [atrSense(chamberPaced,chamberSensed)==1]
  note: SenseStateflow
      | Holds the logic for sensing heart activity and responding to it. The letter code is considered before branching deeper based on the chamber sensed
  note: Function used to determine if in dual mode operation
  note: Bypass used for DXXX modes
  state Pace
    state Charging
      %Discharging Blocking Capacitor C21
      PACE_GND_CTRL = true;
      VENT_PACE_CTRL = false;
      ATR_PACE_CTRL = false;
      if(ActiveChamber == 1)
      ATR_GND_CTRL = true;
      VENT_GND_CTRL = false;
      else
      ATR_GND_CTRL = false;
      VENT_GND_CTRL = true;
      end
      %Sets the Charging of C22
      PACING_REF_PWM = (pulseAmp/5); %pulseAmp
      PACE_CHARGE_CTRL = true;
      send(paceEnd)
    note: Determines chamber to be paced
    state paceAtr
      ATR_PACE_CTRL = true;
    state Discharging
      %Pacing the active chamber
      PACE_CHARGE_CTRL = false;
      PACE_GND_CTRL = true;
      ATR_GND_CTRL = false;
      VENT_GND_CTRL = false;
    state paceVent
      VENT_PACE_CTRL = true;
    note: Setup pins before pacing a chamber
    note: Creates a recharge pulse and charges up the charging
        | capacitor for the next pace
    (default) -> Discharging
    paceAtr -> Charging : after(pulseWidth,msec)
    Discharging -> paceAtr [order 1] : [ActiveChamber == 1]
    paceVent -> Charging : after(pulseWidth,msec)
    Discharging -> paceVent [order 2] : [ActiveChamber == 2]
  note: PaceStateflow
      | Triggered by an event from inside the sense stateflow to immediately discharge the pacing capacitor to the relevant chamber
      | Afterwards it will then trigger the charging state to manipulate the relevant IO to sink the blocking capacitor, and charge the pacing capacitor
      | As IO will be determined by the charging state before leaving this stateflow, the pacing capacitor is always effectively pre-charged
  (junction 278) -> Ventricle [order 1] : [dualSense(chamberPaced,chamberSensed) && ActiveChamber == 1]
  (default) -> INIT
  INIT -> Sense
  Sense -> Pace : paceStart
  (junction 278) -> Sense [order 2]
  Pace -> (junction 278) : paceEnd
  data: a function_input; b function_input; v function_output; v function_output; a function_input; b function_input; a function_input; b function_input; v function_output; Z_ATR_CTRL output; VRP input; atrDetect input boolean; ventDetect input boolean; chamberPaced input; Adjusted input; chamberSensed input; activity input; atrPulseWidth input; atrPulseAmp input; lowerInterval input; upperInterval input; avDelay input; ARP input; ventPulseAmp input; ventPulseWidth input; PVARP input; lowerRate input; upperRate input; PACING_REF_PWM output; Z_VENT_CTRL output; ATR_PACE_CTRL output; VENT_PACE_CTRL output; PACE_GND_CTRL output; ATR_GND_CTRL output; VENT_GND_CTRL output; PACE_CHARGE_CTRL output; R_LED output boolean; B_LED output boolean; ActiveChamber local; iniTime local; pulseWidth local; pulseAmp local
  events: paceStart local FUNCTION_CALL_EVENT; paceEnd local FUNCTION_CALL_EVENT; dischargePace local RISING_EDGE_EVENT; chargePace local RISING_EDGE_EVENT; V_PaceBypass local FUNCTION_CALL_EVENT; AtrSense local FUNCTION_CALL_EVENT; VentSense local FUNCTION_CALL_EVENT; V_Loop local FUNCTION_CALL_EVENT; A_Loop local FUNCTION_CALL_EVENT; Vent_Bypass local FUNCTION_CALL_EVENT
  function v = ventSense(a,b):
    | function  v = ventSense(a,b)
    |     if (a == ChamberPaced.VENTRICLE_P)
    |         v = 1;
    |     elseif (b == ChamberSensed.VENTRICLE_S)
    |         v = 1;
    |     else
    |         v = 0;
    |     end
    | end
  function v = atrSense(a,b):
    | function v = atrSense(a,b)
    |     if (a == ChamberPaced.ATRIUM_P)
    |         v = 1;
    |     elseif (a == ChamberPaced.DUAL_P)
    |         v = 1;
    |     elseif (b == ChamberSensed.ATRIUM_S)
    |         v = 1;
    |     elseif (b == ChamberSensed.DUAL_S)
    |         v = 1;
    |     else
    |         v = 0;
    |     end
    | end
  function v = dualSense(a,b):
    | function v = dualSense(a,b)
    |     if (a == ChamberPaced.DUAL_P)
    |         v = 1;
    |     elseif (b == ChamberSensed.DUAL_S)
    |         v = 1;
    |     else
    |         v = 0;
    |     end
    | end

== stateflow chart Pacemaker/Serial Communication ==
  state SettingParameters
    entry:
    %setting values received from DCM
    Type = 1; %for parameters
    Mode = RX_R(1);
    LRL = RX_R(2);
    URL = RX_R(3);
    AtrialAmp = typecast(RX_R(4:7),'single');
    AtrialPulseWidth = typecast(RX_R(8:11),'single');
    AtrialSensitivity= typecast(RX_R(12:15),'single');
    VentricularAmp = typecast(RX_R(16:19),'single');
    VentricularPulseWidth = typecast(RX_R(20:23),'single');
    VentricularSensitivity = typecast(RX_R(24:27),'single');
    VRP = typecast(RX_R(28:29),'uint16');
    ARP = typecast(RX_R(30:31),'uint16');
    PVARP = typecast(RX_R(32:33),'uint16');
    FixAVDelay = typecast(RX_R(34:35),'uint16');
    MaxSensorRate =  RX_R(36);
    ReactionTime = RX_R(37);
    ResponseFactor = RX_R(38);
    RecoveryTime = RX_R(39);
    ActivityThreshold = RX_R(40);
    Send_DCM(); %Echos back the parameters
  state Init
    entry:
    %Defaults set here
    Mode = 0;
    LRL = 20;
    URL = 80;
    AtrialAmp = 5;
    AtrialPulseWidth = 10;
    VentricularAmp = 4;
    VentricularPulseWidth = 10;
    VRP = 200;
    ARP = 200;
    PVARP =200;
    FixAVDelay = 40;
    MaxSensorRate =  120;
    ReactionTime = 30;
    ResponseFactor = 16;
    RecoveryTime = 5;
    AtrialSensitivity = 3;
    VentricularSensitivity = 3;
    ActivityThreshold = 1;
  state Standby
    %Waiting for DCM
  state WaitForBuffer
    %Waits for new values for the Buffer
  state SendECG
    Type = 0; %for ECG
    Send_DCM();
  SettingParameters -> Standby
  (default) -> Init
  Init -> Standby
  Standby -> (junction 61) : [Status == 0]
  (junction 61) -> SettingParameters [order 2]
  (junction 61) -> WaitForBuffer [order 1] : [RX_R(1) == hex2dec('55')]
  SendECG -> Standby
  WaitForBuffer -> SendECG : [after(20,msec)]
  data: Mode output uint8; LRL output uint8; URL output uint8; AtrialAmp output single; AtrialPulseWidth output single; VentricularAmp output single; VentricularPulseWidth output single; VRP output uint16; RX_R input uint8; Status input uint8; ARP output uint16; PVARP output uint16; FixAVDelay output uint16; MaxSensorRate output uint8; ReactionTime output uint8; ResponseFactor output uint8; RecoveryTime output uint8; AtrialSensitivity output single; VentricularSensitivity output single; ActivityThreshold output uint8; Type output uint8

== stateflow chart Pacemaker/Rate Adaptive/Chart ==
  state Inital
    HeartRate = lowerRate
    activityTime = 0
    noActivityTime = 0
  state SenseActivity
    %decreaseslope is probelm
  state NoActivity
    entry:
    HeartRate = HeartRate - (decreaseSlope/60)*noActivityTime
    exit:
    noActivityTime = elapsed(sec)
  state IncreaseHeartRate
    entry:
    HeartRate = HeartRate + increaseSlope*activityTime
    exit:
    activityTime = elapsed(sec)
  state ReturnToLowerRate
    entry:
    HeartRate = lowerRate
    exit:
    noActivityTime = elapsed(sec)
  state SensorRateAchieved
    entry:
    HeartRate = sensorRate
    exit:
    activityTime = elapsed(sec)
  (default) -> Inital
  Inital -> SenseActivity
  SenseActivity -> (junction 27) [order 1] : [activityThreshold <= 0]
  SenseActivity -> (junction 22) [order 2] : [activityThreshold > 0]
  (junction 54) -> SenseActivity : after(60/HeartRate,sec)
  (junction 27) -> NoActivity [order 2]
  (junction 22) -> IncreaseHeartRate [order 2]
  (junction 22) -> SensorRateAchieved [order 1] : [(HeartRate+increaseSlope*activityTime) >= sensorRate]
  (junction 27) -> ReturnToLowerRate [order 1] : [(HeartRate - (decreaseSlope/60)*noActivityTime) <= lowerRate]
  NoActivity -> (junction 54) : {activityTime=0}
  IncreaseHeartRate -> (junction 54) : {noActivityTime=0}
  ReturnToLowerRate -> (junction 54)
  SensorRateAchieved -> (junction 54)
  data: sensorRate input; increaseSlope input; decreaseSlope input; activityThreshold input; HeartRate output; lowerRate input; activityTime local; noActivityTime local

== stateflow chart Pacemaker/Rate Adaptive/Chart1 ==
  state bufferData
    Activity(2:50) = Activity(1:49)
    Activity(1) = load
    %output = Activity(10)
  note: Used to load data
      | into an array
  (default) -> bufferData
  bufferData -> bufferData : after(10,msec)
  data: load input double =zeros(10,1); Activity output size=50 =zeros(50,1); output local
